simulink model "outputVisualizer"  (R2022a)
settings: Solver=VariableStepAuto  StartTime=0.0  StopTime=10.0  RelTol=1e-3
libraries: sharedtransform x1, uavutilslib x1
settings Model: Creator=Drew Lab Computer 1  LastModifiedBy=Drew Lab Computer 1

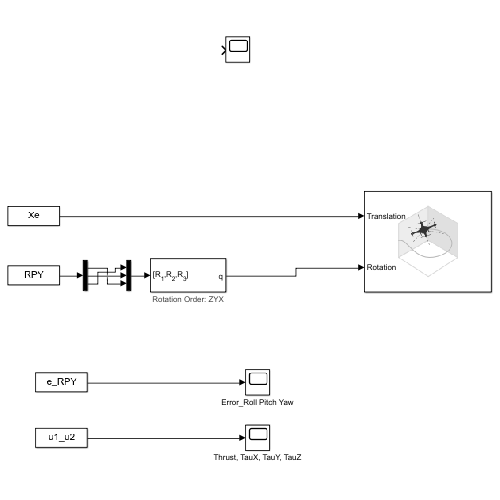
[thumbnail: Simulink's stored preview of the top-level diagram]
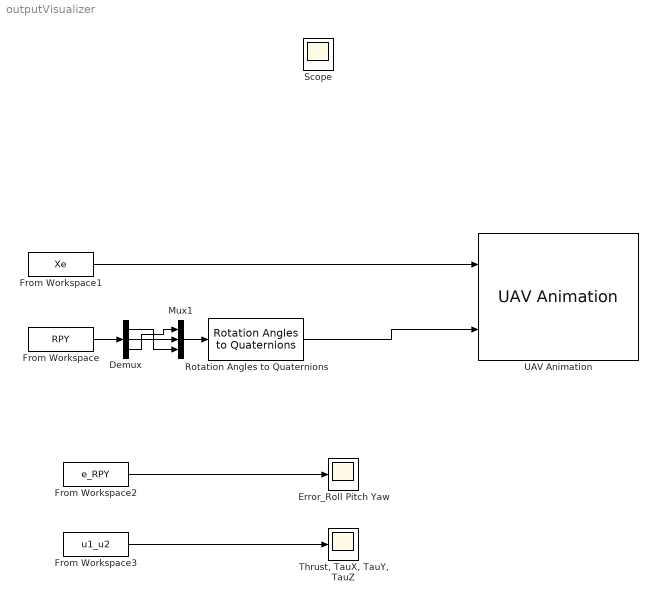
== system outputVisualizer ==
  Demux : Demux  Outputs=3
  Error_Roll Pitch Yaw : Scope
  From Workspace : FromWorkspace  VariableName=RPY
  From Workspace1 : FromWorkspace  VariableName=Xe
  From Workspace2 : FromWorkspace  VariableName=e_RPY
  From Workspace3 : FromWorkspace  VariableName=u1_u2
  Mux1 : Mux  Inputs=3
  Rotation Angles to Quaternions : sharedtransform/Rotation Angles to Quaternions  rotationOrder=ZYX  aMode=aMode
      settings: SourceProductBaseCode=AE,PW,DR,MT,VE
  Scope : Scope
  "Thrust, TauX, TauY, TauZ" : Scope
  UAV Animation : uavutilslib/UAV Animation  UAVType=Multirotor  UAVSize=1  InertialZDirection=Down  SampleTime=1/10000
      settings: SourceProductBaseCode=UV
  wires:
  From Workspace2/1 -> Error_Roll Pitch Yaw/1
  From Workspace3/1 -> "Thrust, TauX, TauY, TauZ"/1
  Rotation Angles to Quaternions/1 -> UAV Animation/2
  From Workspace1/1 -> UAV Animation/1
  From Workspace/1 -> Demux/1
  Mux1/1 -> Rotation Angles to Quaternions/1
  Demux/2 -> Mux1/2
  Demux/1 -> Mux1/3
  Demux/3 -> Mux1/1
